simulink model "disturbances"  (R2020b)
settings: Solver=VariableStepAuto  StartTime=0.0  StopTime=10.0  RelTol=1e-3
values from neighbouring files (symbols this model uses):
  A = [A1,A2,A3,A4,A5,A6,A7,A8]    [dimensions.m]
  Cr = [cr1,cr2,cr3,cr4,cr5,cr6,cr7,cr8]    [dimensions.m]
  Psr = solarFlux/c    (= 4.55648554041e-06)    [main.m]
  Rcp = [rcp1_B,rcp2_B,rcp3_B,rcp4_B,rcp5_B,rcp6_B,rcp7_B,rcp8_B]    [dimensions.m]
  uEarth = 3.986004418e14    (= 398600441800000)    [main.m]
  Un = [un1_B,un2_B,un3_B,un4_B,un5_B,un6_B,un7_B,un8_B]    [dimensions.m]
undefined symbols (not defined in the file or in its folder): A_PB, J_C_P, q0_BI, rcb_B
settings Model: Creator=tjones  LastModifiedBy=tjones

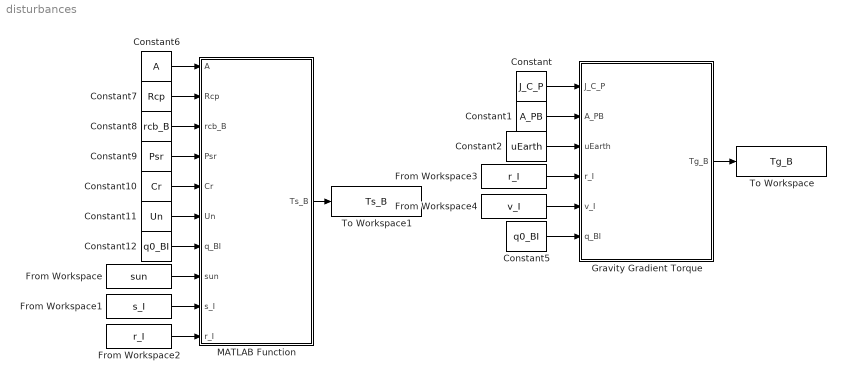
== system disturbances ==
  Constant : Constant  Value=J_C_P
  Constant1 : Constant  Value=A_PB
  Constant10 : Constant  Value=Cr
  Constant11 : Constant  Value=Un
  Constant12 : Constant  Value=q0_BI  OutDataTypeStr=Bus: qBus
  Constant2 : Constant  Value=uEarth
  Constant5 : Constant  Value=q0_BI  OutDataTypeStr=Bus: qBus
  Constant6 : Constant  Value=A
  Constant7 : Constant  Value=Rcp
  Constant8 : Constant  Value=rcb_B
  Constant9 : Constant  Value=Psr
  From Workspace : FromWorkspace  VariableName=sun
  From Workspace1 : FromWorkspace  VariableName=s_I
  From Workspace2 : FromWorkspace  VariableName=r_I
  From Workspace3 : FromWorkspace  VariableName=r_I
  From Workspace4 : FromWorkspace  VariableName=v_I
  Gravity Gradient Torque : MATLAB Function  TreatAsAtomicUnit=on
  MATLAB Function : MATLAB Function  TreatAsAtomicUnit=on
  To Workspace : ToWorkspace  VariableName=Tg_B  SaveFormat=Timeseries  SampleTime=-1
  To Workspace1 : ToWorkspace  VariableName=Ts_B  SaveFormat=Timeseries  SampleTime=-1
  wires:
  Gravity Gradient Torque/1(Tg_B) -> To Workspace/1
  Constant/1 -> Gravity Gradient Torque/1(J_C_P)
  Constant1/1 -> Gravity Gradient Torque/2(A_PB)
  Constant2/1 -> Gravity Gradient Torque/3(uEarth)
  Constant5/1 -> Gravity Gradient Torque/6(q_BI)
  MATLAB Function/1(Ts_B) -> To Workspace1/1
  Constant6/1 -> MATLAB Function/1(A)
  Constant7/1 -> MATLAB Function/2(Rcp)
  Constant8/1 -> MATLAB Function/3(rcb_B)
  Constant9/1 -> MATLAB Function/4(Psr)
  Constant10/1 -> MATLAB Function/5(Cr)
  Constant11/1 -> MATLAB Function/6(Un)
  Constant12/1 -> MATLAB Function/7(q_BI)
  From Workspace/1 -> MATLAB Function/8(sun)
  From Workspace1/1 -> MATLAB Function/9(s_I)
  From Workspace2/1 -> MATLAB Function/10(r_I)
  From Workspace3/1 -> Gravity Gradient Torque/4(r_I)
  From Workspace4/1 -> Gravity Gradient Torque/5(v_I)

== matlab function disturbances/MATLAB Function ==
  data: A input; Ts_B output; Rcp input; rcb_B input; Psr input; Cr input; Un input; q_BI input; sun input; s_I input; r_I input
function Ts_B = solarDisturbance(A, Rcp, rcb_B, Psr, Cr, Un, q_BI, sun, ...
                                 s_I, r_I)

Ts_B = solarTorque(A, Rcp, rcb_B, Psr, Cr, Un, q_BI, sun, s_I, r_I);

== matlab function disturbances/Gravity Gradient Torque ==
  data: J_C_P input; Tg_B output; A_PB input; uEarth input; r_I input; v_I input; q_BI input
function Tg_B = gravityDisturbance(J_C_P, A_PB, uEarth, r_I, v_I, q_BI)

Tg_B = gravityTorque(J_C_P, A_PB, uEarth, r_I, v_I, q_BI);
